simulink model "Rate"  (R2023b)
settings: Solver=VariableStepAuto  StartTime=0.0  StopTime=10.0  RelTol=1e-3
settings Model: Creator=Saif Mohamed  LastModifiedBy=saifg

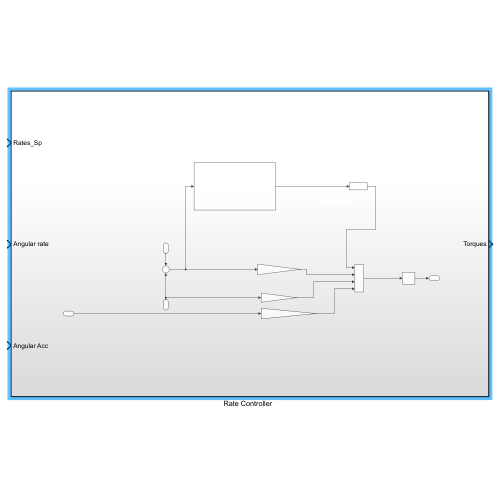
[thumbnail: Simulink's stored preview of the top-level diagram]
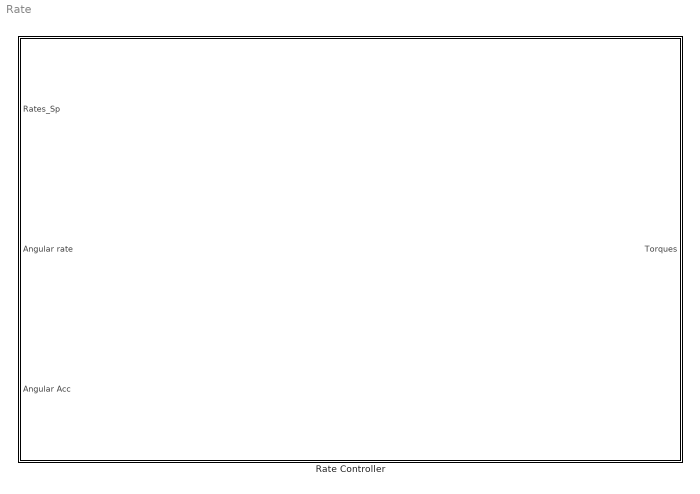
== system Rate ==
  "Rate Controller  " : Subsystem

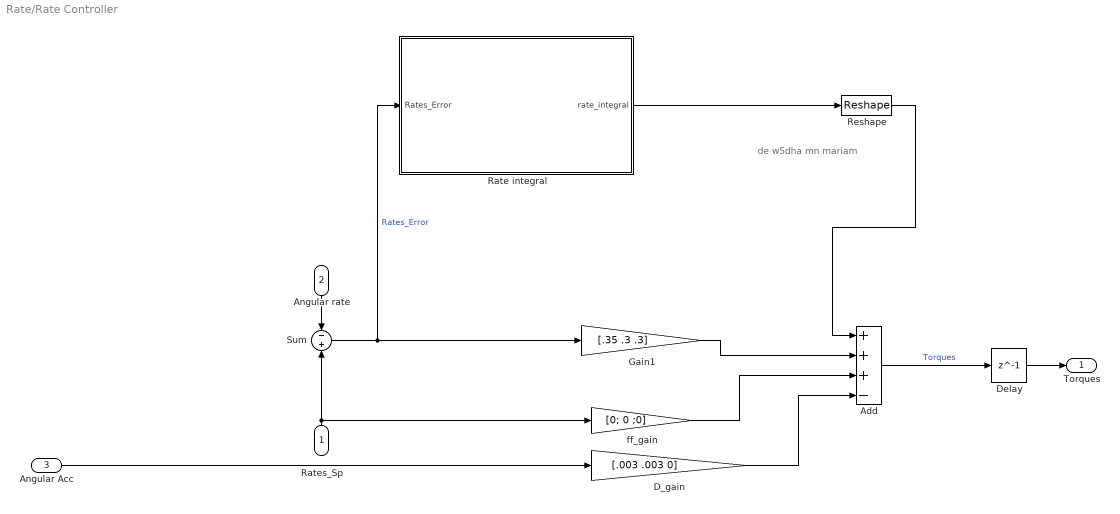
== system Rate/Rate Controller   ==
  note: de w5dha mn mariam
  "Rates_Sp " : Inport
  Angular rate : Inport  Port=2
  Angular Acc : Inport  Port=3
  Add : Sum  Inputs=+++-
  D_gain : Gain  Gain=[.003 .003 0]
  Delay : Delay  DelayLength=1
  Gain1 : Gain  Gain=[.35 .3 .3]
  Rate integral : Subsystem
  Reshape : Reshape  OutputDimensionality=Customize  OutputDimensions=[3]
  Sum : Sum  Inputs=-+
  ff_gain : Gain  Gain=[0; 0 ;0]
  Torques : Outport
  wires:
  "Rates_Sp "/1 -> Sum/2, ff_gain/1
  Add/1 -> Delay/1  "Torques"
  Sum/1 -> Gain1/1, Rate integral/1(Rates_Error)  "Rates_Error"
  Gain1/1 -> Add/2
  ff_gain/1 -> Add/3
  D_gain/1 -> Add/4
  Angular rate/1 -> Sum/1
  Angular Acc/1 -> D_gain/1
  Reshape/1 -> Add/1
  Rate integral/1(rate_integral) -> Reshape/1
  Delay/1 -> Torques/1

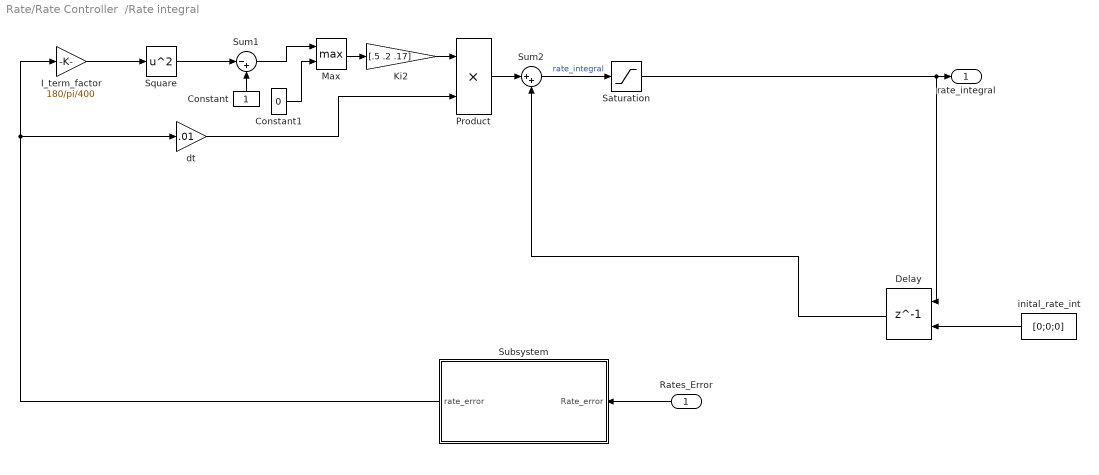
== system Rate/Rate Controller  /Rate integral ==
  Rates_Error : Inport
  Constant : Constant
  Constant1 : Constant  Value=0
  Delay : Delay  DelayLength=1  InitialConditionSource=Input port  InitialCondition=[0;0;0]
      settings: InputPortMap=u0,p4
  I_term_factor : Gain  Gain=180/pi/400
  Ki2 : Gain  Gain=[.5 .2 .17]
  Max : MinMax  Function=max  Inputs=2
  Product : Product
  Saturation : Saturate  UpperLimit=0.3  LowerLimit=-0.3
  Square : Math  Operator=square
  Subsystem : Subsystem
  Sum1 : Sum  Inputs=|-+
  Sum2 : Sum  Inputs=|++
  dt : Gain  Gain=.01
  inital_rate_int : Constant  Value=[0;0;0]
  rate_integral : Outport
  wires:
  Product/1 -> Sum2/1
  Constant/1 -> Sum1/2
  Square/1 -> Sum1/1
  I_term_factor/1 -> Square/1
  dt/1 -> Product/2
  Ki2/1 -> Product/1
  Max/1 -> Ki2/1
  Subsystem/1(rate_error) -> dt/1, I_term_factor/1
  Rates_Error/1 -> Subsystem/1(Rate_error)
  inital_rate_int/1 -> Delay/2
  Sum1/1 -> Max/1
  Constant1/1 -> Max/2
  Sum2/1 -> Saturation/1  "rate_integral"
  Saturation/1 -> Delay/1, rate_integral/1
  Delay/1 -> Sum2/2

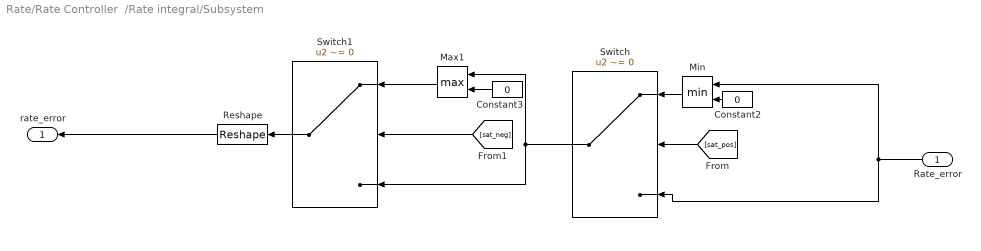
== system Rate/Rate Controller  /Rate integral/Subsystem ==
  Rate_error : Inport
  Constant2 : Constant  Value=0
  Constant3 : Constant  Value=0
  Max1 : MinMax  Function=max  Inputs=2
  Min : MinMax  Inputs=2
  Reshape : Reshape  OutputDimensionality=Customize  OutputDimensions=[3]
  Switch : Switch  Criteria=u2 ~= 0  SaturateOnIntegerOverflow=off  InputSameDT=off
  Switch1 : Switch  Criteria=u2 ~= 0  SaturateOnIntegerOverflow=off  InputSameDT=off
  rate_error : Outport
  wires:
  Min/1 -> Switch/1
  Reshape/1 -> rate_error/1
  Constant2/1 -> Min/2
  [sat_neg] -> Switch1/2
  Rate_error/1 -> Min/1, Switch/3
  [sat_pos] -> Switch/2
  Max1/1 -> Switch1/1
  Constant3/1 -> Max1/2
  Switch1/1 -> Reshape/1
  Switch/1 -> Switch1/3, Max1/1
